simulink model "a0__AM_DSB_FC"  (R2019a)
settings: Solver=VariableStepAuto  StartTime=0.0  StopTime=10.0  RelTol=1e-3
libraries: dsparch4 x1
settings Model: Creator=Thanh_Hai  LastModifiedBy=Thanh_Hai

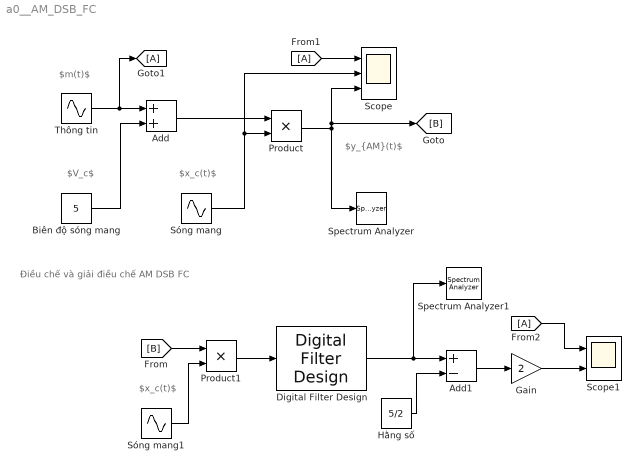
== system a0__AM_DSB_FC ==
  note: Điều chế và giải điều chế AM DSB FC
  note: $V_c$
  note: $x_c(t)$
  note: $m(t)$
  note: $y_{AM}(t)$
  note: $x_c(t)$
  Add : Sum
  Add1 : Sum  Inputs=+-
  Biên độ sóng mang : Constant  Value=5
  Digital Filter Design : dsparch4/Digital Filter Design  mwdsp_browser_bugfix_var=off
  Gain : Gain  Gain=2
  Hằng số : Constant  Value=5/2
  Product : Product
  Product1 : Product
  Scope : Scope  NumInputPorts=3
  Scope1 : Scope  NumInputPorts=2
  Spectrum Analyzer : SpectrumAnalyzer
  Spectrum Analyzer1 : SpectrumAnalyzer
  Sóng mang : Sin  Frequency=2*pi*5000  SampleTime=1/50000
  Sóng mang1 : Sin  Frequency=2*pi*5000  SampleTime=1/50000
  Thông tin : Sin  Amplitude=10  Frequency=2*pi*200  SampleTime=1/50000
  wires:
  Thông tin/1 -> [A], Add/1
  Biên độ sóng mang/1 -> Add/2
  Add/1 -> Product/1
  Sóng mang/1 -> Scope/2, Product/2
  Product/1 -> [B], Scope/3, Spectrum Analyzer/1
  Sóng mang1/1 -> Product1/2
  Product1/1 -> Digital Filter Design/1
  [B] -> Product1/1
  [A] -> Scope/1
  [A] -> Scope1/1
  Digital Filter Design/1 -> Spectrum Analyzer1/1, Add1/1
  Hằng số/1 -> Add1/2
  Add1/1 -> Gain/1
  Gain/1 -> Scope1/2
